simulink model "arte"  (R2013b)
(part 2 of 42)

  Logical2/1 -> pre_dedisp_acc_conv/3(din_valid)
  adder_tree1/1(sync_out) -> pre_dedisp_acc_conv/1(sync_in), Counter6/1
  adder_tree1/2(dout) -> Subsystem3/1(In1)
  Black Box5/2 -> Slice9/1, Slice2/1, Slice5/1, Slice3/1, Slice1/1, Slice4/1, Slice16/1, Slice17/1
  Black Box5/1 -> Convert5/1, Convert46/1
  Convert46/1 -> post_flag_delay/1(sync_in)
  Slice4/1 -> post_flag_delay/2(In1)
  Slice9/1 -> post_flag_delay/3(In2)
  Slice16/1 -> post_flag_delay/4(In3)
  Slice17/1 -> post_flag_delay/5(In4)
  post_flag_delay/2(Out1) -> flag_power/2(din0)
  post_flag_delay/4(Out3) -> flag_power/4(din2)
  post_flag_delay/3(Out2) -> flag_power/3(din1)
  post_flag_delay/1(sync_out) -> flag_power/1(sync_in)
  post_flag_delay/5(Out4) -> flag_power/5(din3)
  flag_power/5(dout3) -> flag_convert/5(In4)
  flag_power/1(sync_out) -> flag_convert/1(sync_in)
  flag_power/4(dout2) -> flag_convert/4(In3)
  flag_power/2(dout0) -> flag_convert/2(In1)
  flag_power/3(dout1) -> flag_convert/3(In2)
  flag_convert/1(sync_out) -> adder_tree1/1(sync)
  flag_convert/3(Out2) -> adder_tree1/3(din2)
  flag_convert/5(Out4) -> adder_tree1/5(din4)
  flag_convert/2(Out1) -> adder_tree1/2(din1)
  flag_convert/4(Out3) -> adder_tree1/4(din3)
  control/17(flag_en) -> [flag_en]
  control/18(flag_num) -> [flag_num]
  control/19(flag_rfi) -> [flag_rfi]
  Counter/1 -> debug/1(addr)
  Reinterpret/1 -> debug/2(data_in)
  control/20(acc_len0) -> [acc_len]
  control/21(acc_len1) -> [acc_len0]
  control/22(acc_len2) -> [acc_len1]
  control/23(acc_len3) -> [acc_len2]
  control/24(acc_len4) -> [acc_len3]
  Reinterpret31/1 -> Concat/1
  Reinterpret24/1 -> Concat/2
  Reinterpret25/1 -> Concat/3
  Reinterpret26/1 -> Concat/4
  Reinterpret4/1 -> Concat1/1
  Reinterpret1/1 -> Concat1/2
  Reinterpret2/1 -> Concat1/3
  Reinterpret3/1 -> Concat1/4
  Reinterpret11/1 -> Concat2/1
  Reinterpret7/1 -> Concat2/2
  Reinterpret8/1 -> Concat2/3
  Reinterpret9/1 -> Concat2/4
  Reinterpret12/1 -> Concat3/1
  Reinterpret5/1 -> Concat3/2
  Reinterpret6/1 -> Concat3/3
  Reinterpret10/1 -> Concat3/4
  Reinterpret16/1 -> Concat4/1
  Reinterpret13/1 -> Concat4/2
  Reinterpret14/1 -> Concat4/3
  Reinterpret15/1 -> Concat4/4
  pipeline30/1 -> sync_tree2/1(In1)
  pipeline53/1 -> m0_tree2/1(In1)
  pipeline27/1 -> m0_en1/1(In1)
  [sd0] -> pipeline13/1(d)
  [m0e0] -> pipeline14/1(d)
  [m0d0] -> Convert1/1
  Convert1/1 -> Reinterpret/1
  pipeline13/1(q) -> Counter/1
  pipeline14/1(q) -> debug/3(we), Counter/2
  pre_dedisp_acc_conv/2(dout) -> pipeline53/1
  pre_dedisp_acc_conv/1(sync_out) -> pipeline30/1
  pre_dedisp_acc_conv/3(dout_valid) -> pipeline27/1
  control/26(rst_dedisp) -> [rst_dedisp]
  control/27(theta1) -> [theta0]
  control/28(theta2) -> [theta1]
  control/29(theta3) -> [theta2]
  control/30(theta4) -> [theta3]
  [acc_len0] -> acc_cntrl5/1(acc_len)
  [sd0] -> acc_cntrl5/2(sync)
  [cnt_rst] -> acc_cntrl5/3(rst)
  acc_cntrl5/1(new_acc) -> pipeline24/1(d), enabled_vacc0/1(new_acc)
  pipeline15/1(q) -> enabled_vacc0/2(din)
  pipeline16/1(q) -> enabled_vacc0/3(din_valid)
  [m0d0] -> Reinterpret18/1
  [m0e0] -> pipeline16/1(d)
  Reinterpret18/1 -> pipeline15/1(d)
  enabled_vacc0/1(dout) -> pre_dedisp_conv0/1(din), Convert2/1
  enabled_vacc0/2(dout_valid) -> pipeline17/1(d), pre_dedisp_conv0/2(din_valid)
  pre_dedisp_conv0/2(dout_valid) -> pre_dedisp_delay0/2(din_valid)
  pre_dedisp_conv0/1(dout) -> pre_dedisp_delay0/1(In1)
  pre_dedisp_delay0/2(dout_valid) -> dedispersor0/3(din_valid)
  pre_dedisp_delay0/1(Out1) -> dedispersor0/2(din)
  [rst_dedisp] -> dedispersor0/1(rst)
  dedispersor0/1(integ_pow) -> post_dedisp_conv0/1(din)
  dedispersor0/2(integ_valid) -> post_dedisp_conv0/2(din_valid)
  post_dedisp_conv0/1(dout) -> post_dedisp_delay0/1(In1)
  post_dedisp_conv0/2(dout_valid) -> post_dedisp_delay0/2(din_valid)
  post_dedisp_delay0/1(Out1) -> Convert3/1, Relational/1, mov_avg0/2(din)
  [rst_dedisp] -> mov_avg0/1(rst)
  mov_avg0/1(dout) -> add_stat0/2
  add_stat0/1 -> Relational/2, Convert4/1
  [theta0] -> add_stat0/1
  Relational/1 -> pipeline42/1
  [rst_detection] -> Register2/2
  Register2/1 -> [detection0]
  Convert2/1 -> Reinterpret17/1
  Reinterpret17/1 -> debug_acc/2(data_in)
  pipeline24/1(q) -> Counter7/1
  pipeline17/1(q) -> Counter7/2, debug_acc/3(we)
  Counter7/1 -> debug_acc/1(addr)
  Counter8/1 -> dedisp0/1(addr)
  post_dedisp_delay0/2(dout_valid) -> Counter8/1, dedisp0/3(we), mov_avg0/3(din_valid)
  Convert3/1 -> Reinterpret19/1
  Reinterpret19/1 -> dedisp0/2(data_in)
  Counter9/1 -> avg0/1(addr)
  mov_avg0/2(dout_valid) -> Counter9/1, avg0/3(we)
  Convert4/1 -> Reinterpret20/1
  Reinterpret20/1 -> avg0/2(data_in)
  Convert5/1 -> beam_rfi_delay/1(sync_in)
  Slice3/1 -> beam_rfi_delay/2(In1)
  Slice5/1 -> beam_rfi_delay/3(In2)
  Slice1/1 -> beam_rfi_delay/4(In3)
  Slice2/1 -> beam_rfi_delay/5(In4)
  beam_rfi_delay/2(Out1) -> beam_rfi_convert/2(In1)
  beam_rfi_delay/3(Out2) -> beam_rfi_convert/3(In2)
  beam_rfi_delay/1(sync_out) -> beam_rfi_convert/1(sync_in)
  beam_rfi_delay/4(Out3) -> beam_rfi_convert/4(In3)
  beam_rfi_delay/5(Out4) -> beam_rfi_convert/5(In4)
  beam_rfi_convert/1(sync_out) -> [beam_sync]
  beam_rfi_convert/2(Out1) -> [beam0]
  beam_rfi_convert/3(Out2) -> [beam1]
  beam_rfi_convert/4(Out3) -> [beam2]
  beam_rfi_convert/5(Out4) -> [beam3]
  rfi_delay/2(Out1) -> rfi_convert/2(In1)
  rfi_delay/3(Out2) -> rfi_convert/3(In2)
  rfi_delay/1(sync_out) -> rfi_convert/1(sync_in)
  rfi_delay/4(Out3) -> rfi_convert/4(In3)
  rfi_delay/5(Out4) -> rfi_convert/5(In4)
  [sync_out3] -> rfi_delay/1(sync_in)
  [fft3_0] -> rfi_delay/2(In1)
  [fft3_1] -> rfi_delay/3(In2)
  [fft3_2] -> rfi_delay/4(In3)
  [fft3_3] -> rfi_delay/5(In4)
  rfi_convert/1(sync_out) -> [rfi_sync]
  rfi_convert/2(Out1) -> [rfi0]
  rfi_convert/3(Out2) -> [rfi1]
  rfi_convert/4(Out3) -> [rfi2]
  rfi_convert/5(Out4) -> [rfi3]
  [tge_rst] -> packetizer/1(rst)
  Mux/1 -> packetizer/2(din)
  [tge_pkt] -> packetizer/3(pkt_len)
  [tge_sleep] -> packetizer/4(sleep_cycle)
  [tge_ip] -> packetizer/5(config_tx_dest_ip)
  Logical1/1 -> packetizer/6(din_valid)
  [tge_port] -> packetizer/7(config_tx_dest_port)
  packetizer/1(tx_data) -> ten_Gbe_v2/2
  packetizer/2(tx_valid) -> ten_Gbe_v2/3
  packetizer/3(tx_dest_ip) -> ten_Gbe_v2/4
  packetizer/4(tx_dest_port) -> ten_Gbe_v2/5
  packetizer/5(tx_eof) -> ten_Gbe_v2/6
  packetizer/6(fifo_full) -> Convert/1
  [acc_len] -> rfi_correlator/1(acc_len)
  [cnt_rst] -> rfi_correlator/2(cnt_rst)
  [rfi_sync] -> rfi_correlator/3(sync_rfi)
  [rfi0] -> rfi_correlator/4(rfi0)
  [rfi1] -> rfi_correlator/5(rfi1)
  [rfi2] -> rfi_correlator/6(rfi2)
  [rfi3] -> rfi_correlator/7(rfi3)
  [beam_sync] -> rfi_correlator/8(sync_beam)
  [beam0] -> rfi_correlator/9(beam0)
  [beam1] -> rfi_correlator/10(beam1)
  [beam2] -> rfi_correlator/11(beam2)
  [beam3] -> rfi_correlator/12(beam3)
  [acc_len] -> rfi_power/1(acc_len)
  [cnt_rst] -> rfi_power/2(cnt_rst)
  [rfi_sync] -> rfi_power/3(rfi_sync)
  [rfi0] -> rfi_power/4(rfi0)
  [rfi1] -> rfi_power/5(rfi1)
  [rfi2] -> rfi_power/6(rfi2)
  [rfi3] -> rfi_power/7(rfi3)
  [beam_sync] -> rfi_power/8(beam_sync)
  [beam0] -> rfi_power/9(beam0)
  [beam1] -> rfi_power/10(beam1)
  [beam2] -> rfi_power/11(beam2)
  [beam3] -> rfi_power/12(beam3)
  rfi_correlator/1(valid_out) -> [rfi_corr_valid]
  rfi_correlator/2(dout0) -> [rfi_corr0]
  rfi_correlator/3(dout1) -> [rfi_corr1]
  rfi_correlator/4(dout2) -> [rfi_corr2]
  rfi_correlator/5(dout3) -> [rfi_corr3]
  rfi_power/1(valid_out) -> [rfi_pow_valid]
  rfi_power/2(dout0) -> [rfi_pow0]
  rfi_power/3(dout1) -> [rfi_pow1]
  rfi_power/4(dout2) -> [rfi_pow2]
  rfi_power/5(dout3) -> [rfi_pow3]
  rfi_power/6(sync_out) -> [rfi_pow_sync]
  Reinterpret30/1 -> Concat11/1
  Reinterpret28/1 -> Concat11/2
  Reinterpret29/1 -> Concat11/3
  Reinterpret32/1 -> Concat11/4
  phase_calc/1(sync_out) -> Counter10/1
  phase_calc/2(dout_valid) -> rfi_flag/3(we), Counter10/2
  phase_calc/3(dout3) -> Reinterpret30/1
  phase_calc/4(dout2) -> Reinterpret28/1
  phase_calc/5(dout1) -> Reinterpret29/1
  phase_calc/6(dout0) -> Reinterpret32/1
  Counter10/1 -> rfi_flag/1(addr)
  Concat11/1 -> rfi_flag/2(data_in)
  rfi_mult/1(data_out) -> Terminator82/1
  pipeline485/1(q) -> Reinterpret95/1
  pipeline476/1(q) -> Counter27/2, rfi_mult/3(we)
  pipeline477/1(q) -> Counter27/1
  pipeline478/1(q) -> Reinterpret92/1
  pipeline480/1(q) -> Reinterpret93/1
  pipeline482/1(q) -> Reinterpret94/1
  Counter27/1 -> rfi_mult/1(addr)
  [rfi_pow_sync] -> pipeline477/1(d)
  [rfi_pow0] -> pipeline485/1(d)
  [rfi_pow1] -> pipeline478/1(d)
  [rfi_pow2] -> pipeline480/1(d)
  [rfi_pow3] -> pipeline482/1(d)
  [rfi_pow_valid] -> pipeline476/1(d)
  pre_phase_delay/3(pow3_out) -> phase_calc/3(rfi_pow3)
  pre_phase_delay/9(pow0_out) -> phase_calc/9(rfi_pow0)
  pre_phase_delay/5(pow2_out) -> phase_calc/5(rfi_pow2)
  pre_phase_delay/8(corr1_out) -> phase_calc/8(rfi_corr1)
  pre_phase_delay/1(sync_out) -> phase_calc/1(sync_in)
  pre_phase_delay/6(corr2_out) -> phase_calc/6(rfi_corr2)
  pre_phase_delay/10(corr0_out) -> phase_calc/10(rfi_corr0)
  pre_phase_delay/4(corr3_out) -> phase_calc/4(rfi_corr3)
  pre_phase_delay/7(pow1_out) -> phase_calc/7(rfi_pow1)
  pre_phase_delay/2(dou_valid) -> phase_calc/2(rfi_pow_valid)
  [rfi_pow_sync] -> pre_phase_delay/1(sync_in)
  [rfi_pow_valid] -> pre_phase_delay/2(din_valid)
  [rfi_pow3] -> pre_phase_delay/3(pow3_in)
  [rfi_corr3] -> pre_phase_delay/4(corr3_in)
  [rfi_pow2] -> pre_phase_delay/5(pow2_in)
  [rfi_corr2] -> pre_phase_delay/6(corr2_in)
  [rfi_pow1] -> pre_phase_delay/7(pow1_in)
  [rfi_corr1] -> pre_phase_delay/8(corr1_in)
  [rfi_pow0] -> pre_phase_delay/9(pow0_in)
  [rfi_corr0] -> pre_phase_delay/10(corr0_in)
  Reinterpret95/1 -> Concat7/1
  Reinterpret94/1 -> Concat7/4
  Reinterpret93/1 -> Concat7/3
  Reinterpret92/1 -> Concat7/2
  Concat7/1 -> rfi_mult/2(data_in)
  rfi_corr/1(data_out) -> Terminator6/1
  pipeline32/1(q) -> Reinterpret27/1
  pipeline25/1(q) -> Counter11/2, rfi_corr/3(we)
  pipeline26/1(q) -> Counter11/1
  pipeline28/1(q) -> Reinterpret21/1
  pipeline29/1(q) -> Reinterpret22/1
  pipeline31/1(q) -> Reinterpret23/1
  Counter11/1 -> rfi_corr/1(addr)
  [rfi_pow_sync] -> pipeline26/1(d)
  [rfi_corr0] -> pipeline32/1(d)
  [rfi_corr1] -> pipeline28/1(d)
  [rfi_corr2] -> pipeline29/1(d)
  [rfi_corr3] -> pipeline31/1(d)
  [rfi_pow_valid] -> pipeline25/1(d)
  Reinterpret27/1 -> Concat8/1
  Reinterpret23/1 -> Concat8/4
  Reinterpret22/1 -> Concat8/3
  Reinterpret21/1 -> Concat8/2
  Concat8/1 -> rfi_corr/2(data_in)
  [acc_len1] -> acc_cntrl6/1(acc_len)
  [sd0] -> acc_cntrl6/2(sync)
  [cnt_rst] -> acc_cntrl6/3(rst)
  acc_cntrl6/1(new_acc) -> enabled_vacc1/1(new_acc)
  pipeline33/1(q) -> enabled_vacc1/2(din)
  pipeline34/1(q) -> enabled_vacc1/3(din_valid)
  [m0d1] -> Reinterpret34/1
  [m0e1] -> pipeline34/1(d)
  Reinterpret34/1 -> pipeline33/1(d)
  enabled_vacc1/1(dout) -> pre_dedisp_conv1/1(din)
  enabled_vacc1/2(dout_valid) -> pre_dedisp_conv1/2(din_valid)
  pre_dedisp_conv1/2(dout_valid) -> pre_dedisp_delay1/2(din_valid)
  pre_dedisp_conv1/1(dout) -> pre_dedisp_delay1/1(In1)
  pre_dedisp_delay1/2(dout_valid) -> dedispersor1/3(din_valid)
  pre_dedisp_delay1/1(Out1) -> dedispersor1/2(din)
  [rst_dedisp] -> dedispersor1/1(rst)
  dedispersor1/1(integ_pow) -> post_dedisp_conv1/1(din)
  dedispersor1/2(integ_valid) -> post_dedisp_conv1/2(din_valid)
  post_dedisp_conv1/1(dout) -> post_dedisp_delay1/1(In1)
  post_dedisp_conv1/2(dout_valid) -> post_dedisp_delay1/2(din_valid)
  post_dedisp_delay1/1(Out1) -> Convert7/1, Relational1/1, mov_avg1/2(din)
  [rst_dedisp] -> mov_avg1/1(rst)
  mov_avg1/1(dout) -> add_stat1/2
  add_stat1/1 -> Relational1/2, Convert8/1
  [theta1] -> add_stat1/1
  Relational1/1 -> pipeline41/1
  [rst_detection] -> Register3/2
  Register3/1 -> [detection1]
  Counter13/1 -> dedisp1/1(addr)
  post_dedisp_delay1/2(dout_valid) -> Counter13/1, dedisp1/3(we), mov_avg1/3(din_valid)
  Convert7/1 -> Reinterpret35/1
  Reinterpret35/1 -> dedisp1/2(data_in)
  Counter14/1 -> avg1/1(addr)
  mov_avg1/2(dout_valid) -> Counter14/1, avg1/3(we)
  Convert8/1 -> Reinterpret36/1
  Reinterpret36/1 -> avg1/2(data_in)
  [acc_len2] -> acc_cntrl7/1(acc_len)
  [sd0] -> acc_cntrl7/2(sync)
  [cnt_rst] -> acc_cntrl7/3(rst)
  acc_cntrl7/1(new_acc) -> enabled_vacc2/1(new_acc)
  pipeline35/1(q) -> enabled_vacc2/2(din)
  pipeline36/1(q) -> enabled_vacc2/3(din_valid)
  [m0d2] -> Reinterpret33/1
  [m0e2] -> pipeline36/1(d)
  Reinterpret33/1 -> pipeline35/1(d)
  enabled_vacc2/1(dout) -> pre_dedisp_conv2/1(din)
  enabled_vacc2/2(dout_valid) -> pre_dedisp_conv2/2(din_valid)
  pre_dedisp_conv2/2(dout_valid) -> pre_dedisp_delay2/2(din_valid)
  pre_dedisp_conv2/1(dout) -> pre_dedisp_delay2/1(In1)
  pre_dedisp_delay2/2(dout_valid) -> dedispersor2/3(din_valid)
  pre_dedisp_delay2/1(Out1) -> dedispersor2/2(din)
  [rst_dedisp] -> dedispersor2/1(rst)
  dedispersor2/1(integ_pow) -> post_dedisp_conv2/1(din)
  dedispersor2/2(integ_valid) -> post_dedisp_conv2/2(din_valid)
  post_dedisp_conv2/1(dout) -> post_dedisp_delay2/1(In1)
  post_dedisp_conv2/2(dout_valid) -> post_dedisp_delay2/2(din_valid)
  post_dedisp_delay2/1(Out1) -> Convert6/1, Relational2/1, mov_avg2/2(din)
  [rst_dedisp] -> mov_avg2/1(rst)
  mov_avg2/1(dout) -> add_stat2/2
  add_stat2/1 -> Relational2/2, Convert9/1
  [theta2] -> add_stat2/1
  Relational2/1 -> pipeline40/1
  [rst_detection] -> Register4/2
  Register4/1 -> [detection2]
  Counter12/1 -> dedisp2/1(addr)
  post_dedisp_delay2/2(dout_valid) -> Counter12/1, dedisp2/3(we), mov_avg2/3(din_valid)
  Convert6/1 -> Reinterpret37/1
  Reinterpret37/1 -> dedisp2/2(data_in)
  Counter15/1 -> avg2/1(addr)
  mov_avg2/2(dout_valid) -> Counter15/1, avg2/3(we)
  Convert9/1 -> Reinterpret38/1
  Reinterpret38/1 -> avg2/2(data_in)
  [acc_len3] -> acc_cntrl8/1(acc_len)
  [sd0] -> acc_cntrl8/2(sync)
  [cnt_rst] -> acc_cntrl8/3(rst)
  acc_cntrl8/1(new_acc) -> enabled_vacc3/1(new_acc)
  pipeline37/1(q) -> enabled_vacc3/2(din)
  pipeline38/1(q) -> enabled_vacc3/3(din_valid)
  [m0d3] -> Reinterpret39/1
  [m0e3] -> pipeline38/1(d)
  Reinterpret39/1 -> pipeline37/1(d)
  enabled_vacc3/1(dout) -> pre_dedisp_conv3/1(din)
  enabled_vacc3/2(dout_valid) -> pre_dedisp_conv3/2(din_valid)
  pre_dedisp_conv3/2(dout_valid) -> pre_dedisp_delay3/2(din_valid)
  pre_dedisp_conv3/1(dout) -> pre_dedisp_delay3/1(In1)
  pre_dedisp_delay3/2(dout_valid) -> dedispersor3/3(din_valid)
  pre_dedisp_delay3/1(Out1) -> dedispersor3/2(din)
  [rst_dedisp] -> dedispersor3/1(rst)
  dedispersor3/1(integ_pow) -> post_dedisp_conv3/1(din)
  dedispersor3/2(integ_valid) -> post_dedisp_conv3/2(din_valid)
  post_dedisp_conv3/1(dout) -> post_dedisp_delay3/1(In1)
  post_dedisp_conv3/2(dout_valid) -> post_dedisp_delay3/2(din_valid)
  post_dedisp_delay3/1(Out1) -> Convert10/1, Relational3/1, mov_avg3/2(din)
  [rst_dedisp] -> mov_avg3/1(rst)
  mov_avg3/1(dout) -> add_stat3/2
  add_stat3/1 -> Relational3/2, Convert11/1
  [theta3] -> add_stat3/1
  Relational3/1 -> pipeline39/1
  [rst_detection] -> Register5/2
  Register5/1 -> [detection3]
  Counter16/1 -> dedisp3/1(addr)
  post_dedisp_delay3/2(dout_valid) -> Counter16/1, dedisp3/3(we), mov_avg3/3(din_valid)
  Convert10/1 -> Reinterpret40/1
  Reinterpret40/1 -> dedisp3/2(data_in)
  Counter17/1 -> avg3/1(addr)
  mov_avg3/2(dout_valid) -> Counter17/1, avg3/3(we)
  Convert11/1 -> Reinterpret41/1
  Reinterpret41/1 -> avg3/2(data_in)
  [detection0] -> Logical3/1
  [detection1] -> Logical3/2
  [detection2] -> Logical3/3
  [detection3] -> Logical3/4
  pipeline39/1 -> Register5/3, Register5/1
  pipeline40/1 -> Register4/3, Register4/1
  pipeline41/1 -> Register3/3, Register3/1
  pipeline42/1 -> Register2/3, Register2/1
  [acc_len4] -> acc_cntrl9/1(acc_len)
  [sd0] -> acc_cntrl9/2(sync)
  [cnt_rst] -> acc_cntrl9/3(rst)
  acc_cntrl9/1(new_acc) -> enabled_vacc4/1(new_acc)
  pipeline43/1(q) -> enabled_vacc4/2(din)
  pipeline45/1(q) -> enabled_vacc4/3(din_valid)
  [m0d4] -> Reinterpret42/1
  [m0e4] -> pipeline45/1(d)
  Reinterpret42/1 -> pipeline43/1(d)
  enabled_vacc4/1(dout) -> pre_dedisp_conv4/1(din)
  enabled_vacc4/2(dout_valid) -> pre_dedisp_conv4/2(din_valid)
  pre_dedisp_conv4/2(dout_valid) -> pre_dedisp_delay4/2(din_valid)
  pre_dedisp_conv4/1(dout) -> pre_dedisp_delay4/1(In1)
  pre_dedisp_delay4/2(dout_valid) -> dedispersor4/3(din_valid)
  pre_dedisp_delay4/1(Out1) -> dedispersor4/2(din)
  [rst_dedisp] -> dedispersor4/1(rst)
  dedispersor4/1(integ_pow) -> post_dedisp_conv4/1(din)
  dedispersor4/2(integ_valid) -> post_dedisp_conv4/2(din_valid)
  post_dedisp_conv4/1(dout) -> post_dedisp_delay4/1(In1)
  post_dedisp_conv4/2(dout_valid) -> post_dedisp_delay4/2(din_valid)
  post_dedisp_delay4/1(Out1) -> Convert12/1, Relational4/1, mov_avg4/2(din)
  [rst_dedisp] -> mov_avg4/1(rst)
  mov_avg4/1(dout) -> add_stat4/2
  add_stat4/1 -> Relational4/2, Convert13/1
  [theta4] -> add_stat4/1
  Relational4/1 -> pipeline46/1
  [rst_detection] -> Register6/2
  Register6/1 -> [detection4]
  Counter18/1 -> dedisp4/1(addr)
  post_dedisp_delay4/2(dout_valid) -> Counter18/1, dedisp4/3(we), mov_avg4/3(din_valid)
  Convert12/1 -> Reinterpret43/1
  Reinterpret43/1 -> dedisp4/2(data_in)
  Counter19/1 -> avg4/1(addr)
  mov_avg4/2(dout_valid) -> Counter19/1, avg4/3(we)
  Convert13/1 -> Reinterpret44/1
  Reinterpret44/1 -> avg4/2(data_in)
  pipeline46/1 -> Register6/3, Register6/1
  [detection4] -> Logical3/5
  control/25(acc_len5) -> [acc_len4]
  control/31(theta5) -> [theta4]
